simulink model "Bujiao_ZuoYe2_1"  (R2020b)
settings: Solver=VariableStepAuto  StartTime=0.0  StopTime=10.0  RelTol=1e-3
settings Model: Creator=19017  LastModifiedBy=19017

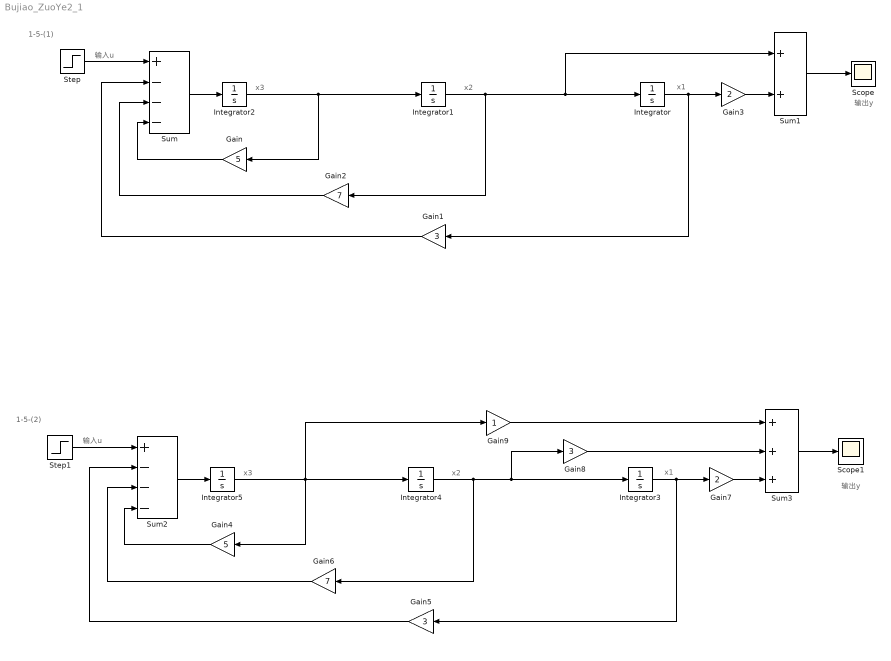
== system Bujiao_ZuoYe2_1 ==
  note: 输出y
  note: 1-5-(1)
  note: 输入u
  note: x3
  note: x2
  note: x1
  note: x2
  note: 输入u
  note: 1-5-(2)
  note: x3
  note: 输出y
  note: x1
  Gain : Gain  Gain=5
  Gain1 : Gain  Gain=3
  Gain2 : Gain  Gain=7
  Gain3 : Gain  Gain=2
  Gain4 : Gain  Gain=5
  Gain5 : Gain  Gain=3
  Gain6 : Gain  Gain=7
  Gain7 : Gain  Gain=2
  Gain8 : Gain  Gain=3
  Gain9 : Gain
  Integrator{,1..5} (6 alike) : Integrator
  Scope : Scope
  Scope1 : Scope
  Step : Step  SampleTime=0
  Step1 : Step  SampleTime=0
  Sum : Sum  Inputs=+---
  Sum1 : Sum
  Sum2 : Sum  Inputs=+---
  Sum3 : Sum  Inputs=+++
  wires:
  Integrator1/1 -> Gain2/1, Sum1/1, Integrator/1
  Integrator2/1 -> Gain/1, Integrator1/1
  Integrator/1 -> Gain3/1, Gain1/1
  Step/1 -> Sum/1
  Sum/1 -> Integrator2/1
  Gain/1 -> Sum/4
  Gain2/1 -> Sum/3
  Gain1/1 -> Sum/2
  Sum1/1 -> Scope/1
  Gain3/1 -> Sum1/2
  Gain5/1 -> Sum2/2
  Sum2/1 -> Integrator5/1
  Integrator4/1 -> Gain6/1, Gain8/1, Integrator3/1
  Gain4/1 -> Sum2/4
  Sum3/1 -> Scope1/1
  Integrator3/1 -> Gain7/1, Gain5/1
  Step1/1 -> Sum2/1
  Gain6/1 -> Sum2/3
  Integrator5/1 -> Gain4/1, Gain9/1, Integrator4/1
  Gain7/1 -> Sum3/3
  Gain8/1 -> Sum3/2
  Gain9/1 -> Sum3/1
